simulink model "empirical_cell_twaice_balancing"  (R2024b)
settings: Solver=FixedStepAuto  StartTime=0.0  StopTime=inf  FixedStep=1  RelTol=1e-3
values from neighbouring files (symbols this model uses):
  act = 1    [RunMe_TWAICE_Cell_Model_Farasis_P75_75Ah_v8_1_3.m]
  lic_no = fin_convert(Prod_lic)    [RunMe_TWAICE_Cell_Model_Farasis_P75_75Ah_v8_1_3.m]
  Ts = 1    [RunMe_TWAICE_Cell_Model_Farasis_P75_75Ah_v8_1_3.m]
undefined symbols (not defined in the file or in its folder): DWORK0, DWORK1, DWORK10, DWORK11, DWORK12, DWORK13, DWORK14, DWORK15, DWORK16, DWORK17, DWORK18, DWORK19, DWORK2, DWORK20, DWORK22, DWORK23, DWORK24, DWORK25, DWORK26, DWORK27, DWORK28, DWORK29, DWORK3, DWORK30, DWORK31, DWORK32, DWORK33, DWORK34, DWORK35, DWORK36, DWORK4, DWORK5, DWORK6, DWORK7, DWORK8, DWORK9, SOHc_init, SOHr_init
libraries: fl_lib x73, nesl_utility x32, ee_lib x8
(part 4 of 4)

== system empirical_cell_twaice_balancing/Cell 4/SOC coloumb counting1/__OutputSSForSFun__ ==
  __UniqueInportName__1__ : Inport
  SOC : Outport  VectorParamsAs1DForOutWhenUnconnected=off
  wires:
  __UniqueInportName__1__/1 -> SOC/1

== system empirical_cell_twaice_balancing/Cell 5/ETA Model 1/__InputSSForSFun__ ==
  "Current " : Inport  OutDataTypeStr=double  PortDimensions=1
  T_ambient / °C : Inport  Port=2  OutDataTypeStr=double  PortDimensions=1
  SOHc_init : Inport  Port=3
  SOHr_init : Inport  Port=4
  SOC_init : Inport  Port=5
  T_init : Inport  Port=6
  SOC_in : Inport  Port=7
  SOH : Inport  Port=8
  Constant : Constant  Value=0
  Constant1 : Constant  Value=0
  temporaryBusSelectName_2 : BusSelector  OutputSignals=SOHc,SOHr
  __UniqueOutportName__1__ : Outport  VectorParamsAs1DForOutWhenUnconnected=off
  __UniqueOutportName__2__ : Outport  Port=2  VectorParamsAs1DForOutWhenUnconnected=off
  __UniqueOutportName__3__ : Outport  Port=3  VectorParamsAs1DForOutWhenUnconnected=off
  __UniqueOutportName__4__ : Outport  Port=4  VectorParamsAs1DForOutWhenUnconnected=off
  __UniqueOutportName__5__ : Outport  Port=5  VectorParamsAs1DForOutWhenUnconnected=off
  __UniqueOutportName__6__ : Outport  Port=6  VectorParamsAs1DForOutWhenUnconnected=off
  __UniqueOutportName__7__ : Outport  Port=7  VectorParamsAs1DForOutWhenUnconnected=off
  __UniqueOutportName__8__ : Outport  Port=8  VectorParamsAs1DForOutWhenUnconnected=off
  __UniqueOutportName__9__ : Outport  Port=9  VectorParamsAs1DForOutWhenUnconnected=off
  __UniqueOutportName__10__ : Outport  Port=10  VectorParamsAs1DForOutWhenUnconnected=off
  __UniqueOutportName__11__ : Outport  Port=11  VectorParamsAs1DForOutWhenUnconnected=off
  wires:
  SOH/1 -> temporaryBusSelectName_2/1
  "Current "/1 -> __UniqueOutportName__1__/1
  T_ambient / °C/1 -> __UniqueOutportName__2__/1
  SOHc_init/1 -> __UniqueOutportName__5__/1
  SOHr_init/1 -> __UniqueOutportName__6__/1
  SOC_init/1 -> __UniqueOutportName__7__/1
  T_init/1 -> __UniqueOutportName__8__/1
  SOC_in/1 -> __UniqueOutportName__9__/1
  temporaryBusSelectName_2/1 -> __UniqueOutportName__10__/1  "<SOHc>"
  temporaryBusSelectName_2/2 -> __UniqueOutportName__11__/1  "<SOHr>"
  Constant/1 -> __UniqueOutportName__3__/1
  Constant1/1 -> __UniqueOutportName__4__/1

== system empirical_cell_twaice_balancing/Cell 5/ETA Model 1/__OutputSSForSFun__ ==
  __UniqueInportName__1__ : Inport
  __UniqueInportName__2__ : Inport  Port=2
  __UniqueInportName__3__ : Inport  Port=3
  __UniqueInportName__4__ : Inport  Port=4
  __UniqueInportName__5__ : Inport  Port=5
  __UniqueInportName__6__ : Inport  Port=6
  __UniqueInportName__7__ : Inport  Port=7
  __UniqueInportName__8__ : Inport  Port=8
  __UniqueInportName__9__ : Inport  Port=9
  Current / A : Outport  OutDataTypeStr=double  PortDimensions=1
  Voltage / V : Outport  Port=2  OutDataTypeStr=double  PortDimensions=1
  SOC / 0..1 : Outport  Port=3  OutDataTypeStr=double  PortDimensions=1
  SOHc / 0..1 : Outport  Port=4  OutDataTypeStr=double  PortDimensions=1
  T_sim / °C : Outport  Port=5  OutDataTypeStr=double  PortDimensions=1
  Generated Heat / W : Outport  Port=6  OutDataTypeStr=double  PortDimensions=1
  SOHr / 1 : Outport  Port=7  OutDataTypeStr=double  PortDimensions=1
  Power_sim / W : Outport  Port=8  OutDataTypeStr=double  PortDimensions=1
  total_Ah : Outport  Port=9
  wires:
  __UniqueInportName__1__/1 -> Current / A/1  "I"
  __UniqueInportName__2__/1 -> Voltage / V/1  "U"
  __UniqueInportName__3__/1 -> SOC / 0..1/1
  __UniqueInportName__4__/1 -> SOHc / 0..1/1  "SOHc"
  __UniqueInportName__5__/1 -> T_sim / °C/1  "simulated Temperature"
  __UniqueInportName__6__/1 -> Generated Heat / W/1
  __UniqueInportName__7__/1 -> SOHr / 1/1  "SOHr"
  __UniqueInportName__8__/1 -> Power_sim / W/1
  __UniqueInportName__9__/1 -> total_Ah/1  "total_Ah"

== system empirical_cell_twaice_balancing/Cell 5/SOC coloumb counting1/__InputSSForSFun__ ==
  SOC_init : Inport
  T_init : Inport  Port=2
  I [A] : Inport  Port=3
  SOHc : Inport  Port=4
  Tcell : Inport  Port=5
  __UniqueOutportName__1__ : Outport  VectorParamsAs1DForOutWhenUnconnected=off
  __UniqueOutportName__2__ : Outport  Port=2  VectorParamsAs1DForOutWhenUnconnected=off
  __UniqueOutportName__3__ : Outport  Port=3  VectorParamsAs1DForOutWhenUnconnected=off
  __UniqueOutportName__4__ : Outport  Port=4  VectorParamsAs1DForOutWhenUnconnected=off
  __UniqueOutportName__5__ : Outport  Port=5  VectorParamsAs1DForOutWhenUnconnected=off
  wires:
  SOC_init/1 -> __UniqueOutportName__1__/1
  T_init/1 -> __UniqueOutportName__2__/1
  I [A]/1 -> __UniqueOutportName__3__/1
  SOHc/1 -> __UniqueOutportName__4__/1
  Tcell/1 -> __UniqueOutportName__5__/1

== system empirical_cell_twaice_balancing/Cell 5/SOC coloumb counting1/__OutputSSForSFun__ ==
  __UniqueInportName__1__ : Inport
  SOC : Outport  VectorParamsAs1DForOutWhenUnconnected=off
  wires:
  __UniqueInportName__1__/1 -> SOC/1

== system empirical_cell_twaice_balancing/Cell 6/ETA Model 1/__InputSSForSFun__ ==
  "Current " : Inport  OutDataTypeStr=double  PortDimensions=1
  T_ambient / °C : Inport  Port=2  OutDataTypeStr=double  PortDimensions=1
  SOHc_init : Inport  Port=3
  SOHr_init : Inport  Port=4
  SOC_init : Inport  Port=5
  T_init : Inport  Port=6
  SOC_in : Inport  Port=7
  SOH : Inport  Port=8
  Constant : Constant  Value=0
  Constant1 : Constant  Value=0
  temporaryBusSelectName_2 : BusSelector  OutputSignals=SOHc,SOHr
  __UniqueOutportName__1__ : Outport  VectorParamsAs1DForOutWhenUnconnected=off
  __UniqueOutportName__2__ : Outport  Port=2  VectorParamsAs1DForOutWhenUnconnected=off
  __UniqueOutportName__3__ : Outport  Port=3  VectorParamsAs1DForOutWhenUnconnected=off
  __UniqueOutportName__4__ : Outport  Port=4  VectorParamsAs1DForOutWhenUnconnected=off
  __UniqueOutportName__5__ : Outport  Port=5  VectorParamsAs1DForOutWhenUnconnected=off
  __UniqueOutportName__6__ : Outport  Port=6  VectorParamsAs1DForOutWhenUnconnected=off
  __UniqueOutportName__7__ : Outport  Port=7  VectorParamsAs1DForOutWhenUnconnected=off
  __UniqueOutportName__8__ : Outport  Port=8  VectorParamsAs1DForOutWhenUnconnected=off
  __UniqueOutportName__9__ : Outport  Port=9  VectorParamsAs1DForOutWhenUnconnected=off
  __UniqueOutportName__10__ : Outport  Port=10  VectorParamsAs1DForOutWhenUnconnected=off
  __UniqueOutportName__11__ : Outport  Port=11  VectorParamsAs1DForOutWhenUnconnected=off
  wires:
  SOH/1 -> temporaryBusSelectName_2/1
  "Current "/1 -> __UniqueOutportName__1__/1
  T_ambient / °C/1 -> __UniqueOutportName__2__/1
  SOHc_init/1 -> __UniqueOutportName__5__/1
  SOHr_init/1 -> __UniqueOutportName__6__/1
  SOC_init/1 -> __UniqueOutportName__7__/1
  T_init/1 -> __UniqueOutportName__8__/1
  SOC_in/1 -> __UniqueOutportName__9__/1
  temporaryBusSelectName_2/1 -> __UniqueOutportName__10__/1  "<SOHc>"
  temporaryBusSelectName_2/2 -> __UniqueOutportName__11__/1  "<SOHr>"
  Constant/1 -> __UniqueOutportName__3__/1
  Constant1/1 -> __UniqueOutportName__4__/1

== system empirical_cell_twaice_balancing/Cell 6/ETA Model 1/__OutputSSForSFun__ ==
  __UniqueInportName__1__ : Inport
  __UniqueInportName__2__ : Inport  Port=2
  __UniqueInportName__3__ : Inport  Port=3
  __UniqueInportName__4__ : Inport  Port=4
  __UniqueInportName__5__ : Inport  Port=5
  __UniqueInportName__6__ : Inport  Port=6
  __UniqueInportName__7__ : Inport  Port=7
  __UniqueInportName__8__ : Inport  Port=8
  __UniqueInportName__9__ : Inport  Port=9
  Current / A : Outport  OutDataTypeStr=double  PortDimensions=1
  Voltage / V : Outport  Port=2  OutDataTypeStr=double  PortDimensions=1
  SOC / 0..1 : Outport  Port=3  OutDataTypeStr=double  PortDimensions=1
  SOHc / 0..1 : Outport  Port=4  OutDataTypeStr=double  PortDimensions=1
  T_sim / °C : Outport  Port=5  OutDataTypeStr=double  PortDimensions=1
  Generated Heat / W : Outport  Port=6  OutDataTypeStr=double  PortDimensions=1
  SOHr / 1 : Outport  Port=7  OutDataTypeStr=double  PortDimensions=1
  Power_sim / W : Outport  Port=8  OutDataTypeStr=double  PortDimensions=1
  total_Ah : Outport  Port=9
  wires:
  __UniqueInportName__1__/1 -> Current / A/1  "I"
  __UniqueInportName__2__/1 -> Voltage / V/1  "U"
  __UniqueInportName__3__/1 -> SOC / 0..1/1
  __UniqueInportName__4__/1 -> SOHc / 0..1/1  "SOHc"
  __UniqueInportName__5__/1 -> T_sim / °C/1  "simulated Temperature"
  __UniqueInportName__6__/1 -> Generated Heat / W/1
  __UniqueInportName__7__/1 -> SOHr / 1/1  "SOHr"
  __UniqueInportName__8__/1 -> Power_sim / W/1
  __UniqueInportName__9__/1 -> total_Ah/1  "total_Ah"

== system empirical_cell_twaice_balancing/Cell 6/SOC coloumb counting1/__InputSSForSFun__ ==
  SOC_init : Inport
  T_init : Inport  Port=2
  I [A] : Inport  Port=3
  SOHc : Inport  Port=4
  Tcell : Inport  Port=5
  __UniqueOutportName__1__ : Outport  VectorParamsAs1DForOutWhenUnconnected=off
  __UniqueOutportName__2__ : Outport  Port=2  VectorParamsAs1DForOutWhenUnconnected=off
  __UniqueOutportName__3__ : Outport  Port=3  VectorParamsAs1DForOutWhenUnconnected=off
  __UniqueOutportName__4__ : Outport  Port=4  VectorParamsAs1DForOutWhenUnconnected=off
  __UniqueOutportName__5__ : Outport  Port=5  VectorParamsAs1DForOutWhenUnconnected=off
  wires:
  SOC_init/1 -> __UniqueOutportName__1__/1
  T_init/1 -> __UniqueOutportName__2__/1
  I [A]/1 -> __UniqueOutportName__3__/1
  SOHc/1 -> __UniqueOutportName__4__/1
  Tcell/1 -> __UniqueOutportName__5__/1

== system empirical_cell_twaice_balancing/Cell 6/SOC coloumb counting1/__OutputSSForSFun__ ==
  __UniqueInportName__1__ : Inport
  SOC : Outport  VectorParamsAs1DForOutWhenUnconnected=off
  wires:
  __UniqueInportName__1__/1 -> SOC/1

== system empirical_cell_twaice_balancing/Cell 7/ETA Model 1/__InputSSForSFun__ ==
  "Current " : Inport  OutDataTypeStr=double  PortDimensions=1
  T_ambient / °C : Inport  Port=2  OutDataTypeStr=double  PortDimensions=1
  SOHc_init : Inport  Port=3
  SOHr_init : Inport  Port=4
  SOC_init : Inport  Port=5
  T_init : Inport  Port=6
  SOC_in : Inport  Port=7
  SOH : Inport  Port=8
  Constant : Constant  Value=0
  Constant1 : Constant  Value=0
  temporaryBusSelectName_2 : BusSelector  OutputSignals=SOHc,SOHr
  __UniqueOutportName__1__ : Outport  VectorParamsAs1DForOutWhenUnconnected=off
  __UniqueOutportName__2__ : Outport  Port=2  VectorParamsAs1DForOutWhenUnconnected=off
  __UniqueOutportName__3__ : Outport  Port=3  VectorParamsAs1DForOutWhenUnconnected=off
  __UniqueOutportName__4__ : Outport  Port=4  VectorParamsAs1DForOutWhenUnconnected=off
  __UniqueOutportName__5__ : Outport  Port=5  VectorParamsAs1DForOutWhenUnconnected=off
  __UniqueOutportName__6__ : Outport  Port=6  VectorParamsAs1DForOutWhenUnconnected=off
  __UniqueOutportName__7__ : Outport  Port=7  VectorParamsAs1DForOutWhenUnconnected=off
  __UniqueOutportName__8__ : Outport  Port=8  VectorParamsAs1DForOutWhenUnconnected=off
  __UniqueOutportName__9__ : Outport  Port=9  VectorParamsAs1DForOutWhenUnconnected=off
  __UniqueOutportName__10__ : Outport  Port=10  VectorParamsAs1DForOutWhenUnconnected=off
  __UniqueOutportName__11__ : Outport  Port=11  VectorParamsAs1DForOutWhenUnconnected=off
  wires:
  SOH/1 -> temporaryBusSelectName_2/1
  "Current "/1 -> __UniqueOutportName__1__/1
  T_ambient / °C/1 -> __UniqueOutportName__2__/1
  SOHc_init/1 -> __UniqueOutportName__5__/1
  SOHr_init/1 -> __UniqueOutportName__6__/1
  SOC_init/1 -> __UniqueOutportName__7__/1
  T_init/1 -> __UniqueOutportName__8__/1
  SOC_in/1 -> __UniqueOutportName__9__/1
  temporaryBusSelectName_2/1 -> __UniqueOutportName__10__/1  "<SOHc>"
  temporaryBusSelectName_2/2 -> __UniqueOutportName__11__/1  "<SOHr>"
  Constant/1 -> __UniqueOutportName__3__/1
  Constant1/1 -> __UniqueOutportName__4__/1

== system empirical_cell_twaice_balancing/Cell 7/ETA Model 1/__OutputSSForSFun__ ==
  __UniqueInportName__1__ : Inport
  __UniqueInportName__2__ : Inport  Port=2
  __UniqueInportName__3__ : Inport  Port=3
  __UniqueInportName__4__ : Inport  Port=4
  __UniqueInportName__5__ : Inport  Port=5
  __UniqueInportName__6__ : Inport  Port=6
  __UniqueInportName__7__ : Inport  Port=7
  __UniqueInportName__8__ : Inport  Port=8
  __UniqueInportName__9__ : Inport  Port=9
  Current / A : Outport  OutDataTypeStr=double  PortDimensions=1
  Voltage / V : Outport  Port=2  OutDataTypeStr=double  PortDimensions=1
  SOC / 0..1 : Outport  Port=3  OutDataTypeStr=double  PortDimensions=1
  SOHc / 0..1 : Outport  Port=4  OutDataTypeStr=double  PortDimensions=1
  T_sim / °C : Outport  Port=5  OutDataTypeStr=double  PortDimensions=1
  Generated Heat / W : Outport  Port=6  OutDataTypeStr=double  PortDimensions=1
  SOHr / 1 : Outport  Port=7  OutDataTypeStr=double  PortDimensions=1
  Power_sim / W : Outport  Port=8  OutDataTypeStr=double  PortDimensions=1
  total_Ah : Outport  Port=9
  wires:
  __UniqueInportName__1__/1 -> Current / A/1  "I"
  __UniqueInportName__2__/1 -> Voltage / V/1  "U"
  __UniqueInportName__3__/1 -> SOC / 0..1/1
  __UniqueInportName__4__/1 -> SOHc / 0..1/1  "SOHc"
  __UniqueInportName__5__/1 -> T_sim / °C/1  "simulated Temperature"
  __UniqueInportName__6__/1 -> Generated Heat / W/1
  __UniqueInportName__7__/1 -> SOHr / 1/1  "SOHr"
  __UniqueInportName__8__/1 -> Power_sim / W/1
  __UniqueInportName__9__/1 -> total_Ah/1  "total_Ah"

== system empirical_cell_twaice_balancing/Cell 7/SOC coloumb counting1/__InputSSForSFun__ ==
  SOC_init : Inport
  T_init : Inport  Port=2
  I [A] : Inport  Port=3
  SOHc : Inport  Port=4
  Tcell : Inport  Port=5
  __UniqueOutportName__1__ : Outport  VectorParamsAs1DForOutWhenUnconnected=off
  __UniqueOutportName__2__ : Outport  Port=2  VectorParamsAs1DForOutWhenUnconnected=off
  __UniqueOutportName__3__ : Outport  Port=3  VectorParamsAs1DForOutWhenUnconnected=off
  __UniqueOutportName__4__ : Outport  Port=4  VectorParamsAs1DForOutWhenUnconnected=off
  __UniqueOutportName__5__ : Outport  Port=5  VectorParamsAs1DForOutWhenUnconnected=off
  wires:
  SOC_init/1 -> __UniqueOutportName__1__/1
  T_init/1 -> __UniqueOutportName__2__/1
  I [A]/1 -> __UniqueOutportName__3__/1
  SOHc/1 -> __UniqueOutportName__4__/1
  Tcell/1 -> __UniqueOutportName__5__/1

== system empirical_cell_twaice_balancing/Cell 7/SOC coloumb counting1/__OutputSSForSFun__ ==
  __UniqueInportName__1__ : Inport
  SOC : Outport  VectorParamsAs1DForOutWhenUnconnected=off
  wires:
  __UniqueInportName__1__/1 -> SOC/1

== system empirical_cell_twaice_balancing/Cell 8/ETA Model 1/__InputSSForSFun__ ==
  "Current " : Inport  OutDataTypeStr=double  PortDimensions=1
  T_ambient / °C : Inport  Port=2  OutDataTypeStr=double  PortDimensions=1
  SOHc_init : Inport  Port=3
  SOHr_init : Inport  Port=4
  SOC_init : Inport  Port=5
  T_init : Inport  Port=6
  SOC_in : Inport  Port=7
  SOH : Inport  Port=8
  Constant : Constant  Value=0
  Constant1 : Constant  Value=0
  temporaryBusSelectName_2 : BusSelector  OutputSignals=SOHc,SOHr
  __UniqueOutportName__1__ : Outport  VectorParamsAs1DForOutWhenUnconnected=off
  __UniqueOutportName__2__ : Outport  Port=2  VectorParamsAs1DForOutWhenUnconnected=off
  __UniqueOutportName__3__ : Outport  Port=3  VectorParamsAs1DForOutWhenUnconnected=off
  __UniqueOutportName__4__ : Outport  Port=4  VectorParamsAs1DForOutWhenUnconnected=off
  __UniqueOutportName__5__ : Outport  Port=5  VectorParamsAs1DForOutWhenUnconnected=off
  __UniqueOutportName__6__ : Outport  Port=6  VectorParamsAs1DForOutWhenUnconnected=off
  __UniqueOutportName__7__ : Outport  Port=7  VectorParamsAs1DForOutWhenUnconnected=off
  __UniqueOutportName__8__ : Outport  Port=8  VectorParamsAs1DForOutWhenUnconnected=off
  __UniqueOutportName__9__ : Outport  Port=9  VectorParamsAs1DForOutWhenUnconnected=off
  __UniqueOutportName__10__ : Outport  Port=10  VectorParamsAs1DForOutWhenUnconnected=off
  __UniqueOutportName__11__ : Outport  Port=11  VectorParamsAs1DForOutWhenUnconnected=off
  wires:
  SOH/1 -> temporaryBusSelectName_2/1
  "Current "/1 -> __UniqueOutportName__1__/1
  T_ambient / °C/1 -> __UniqueOutportName__2__/1
  SOHc_init/1 -> __UniqueOutportName__5__/1
  SOHr_init/1 -> __UniqueOutportName__6__/1
  SOC_init/1 -> __UniqueOutportName__7__/1
  T_init/1 -> __UniqueOutportName__8__/1
  SOC_in/1 -> __UniqueOutportName__9__/1
  temporaryBusSelectName_2/1 -> __UniqueOutportName__10__/1  "<SOHc>"
  temporaryBusSelectName_2/2 -> __UniqueOutportName__11__/1  "<SOHr>"
  Constant/1 -> __UniqueOutportName__3__/1
  Constant1/1 -> __UniqueOutportName__4__/1

== system empirical_cell_twaice_balancing/Cell 8/ETA Model 1/__OutputSSForSFun__ ==
  __UniqueInportName__1__ : Inport
  __UniqueInportName__2__ : Inport  Port=2
  __UniqueInportName__3__ : Inport  Port=3
  __UniqueInportName__4__ : Inport  Port=4
  __UniqueInportName__5__ : Inport  Port=5
  __UniqueInportName__6__ : Inport  Port=6
  __UniqueInportName__7__ : Inport  Port=7
  __UniqueInportName__8__ : Inport  Port=8
  __UniqueInportName__9__ : Inport  Port=9
  Current / A : Outport  OutDataTypeStr=double  PortDimensions=1
  Voltage / V : Outport  Port=2  OutDataTypeStr=double  PortDimensions=1
  SOC / 0..1 : Outport  Port=3  OutDataTypeStr=double  PortDimensions=1
  SOHc / 0..1 : Outport  Port=4  OutDataTypeStr=double  PortDimensions=1
  T_sim / °C : Outport  Port=5  OutDataTypeStr=double  PortDimensions=1
  Generated Heat / W : Outport  Port=6  OutDataTypeStr=double  PortDimensions=1
  SOHr / 1 : Outport  Port=7  OutDataTypeStr=double  PortDimensions=1
  Power_sim / W : Outport  Port=8  OutDataTypeStr=double  PortDimensions=1
  total_Ah : Outport  Port=9
  wires:
  __UniqueInportName__1__/1 -> Current / A/1  "I"
  __UniqueInportName__2__/1 -> Voltage / V/1  "U"
  __UniqueInportName__3__/1 -> SOC / 0..1/1
  __UniqueInportName__4__/1 -> SOHc / 0..1/1  "SOHc"
  __UniqueInportName__5__/1 -> T_sim / °C/1  "simulated Temperature"
  __UniqueInportName__6__/1 -> Generated Heat / W/1
  __UniqueInportName__7__/1 -> SOHr / 1/1  "SOHr"
  __UniqueInportName__8__/1 -> Power_sim / W/1
  __UniqueInportName__9__/1 -> total_Ah/1  "total_Ah"

== system empirical_cell_twaice_balancing/Cell 8/SOC coloumb counting1/__InputSSForSFun__ ==
  SOC_init : Inport
  T_init : Inport  Port=2
  I [A] : Inport  Port=3
  SOHc : Inport  Port=4
  Tcell : Inport  Port=5
  __UniqueOutportName__1__ : Outport  VectorParamsAs1DForOutWhenUnconnected=off
  __UniqueOutportName__2__ : Outport  Port=2  VectorParamsAs1DForOutWhenUnconnected=off
  __UniqueOutportName__3__ : Outport  Port=3  VectorParamsAs1DForOutWhenUnconnected=off
  __UniqueOutportName__4__ : Outport  Port=4  VectorParamsAs1DForOutWhenUnconnected=off
  __UniqueOutportName__5__ : Outport  Port=5  VectorParamsAs1DForOutWhenUnconnected=off
  wires:
  SOC_init/1 -> __UniqueOutportName__1__/1
  T_init/1 -> __UniqueOutportName__2__/1
  I [A]/1 -> __UniqueOutportName__3__/1
  SOHc/1 -> __UniqueOutportName__4__/1
  Tcell/1 -> __UniqueOutportName__5__/1

== system empirical_cell_twaice_balancing/Cell 8/SOC coloumb counting1/__OutputSSForSFun__ ==
  __UniqueInportName__1__ : Inport
  SOC : Outport  VectorParamsAs1DForOutWhenUnconnected=off
  wires:
  __UniqueInportName__1__/1 -> SOC/1
